simulink model "Bremsvorgang"  (R2023a)
settings: Solver=VariableStepAuto  StartTime=0.0  StopTime=10.0  RelTol=1e-3
settings Model: Creator=victoriastrobel  LastModifiedBy=victoriastrobel

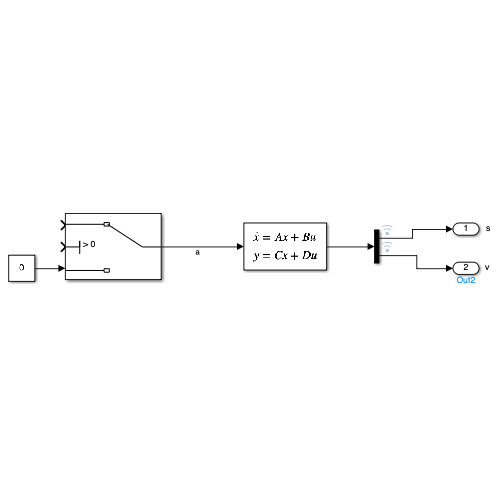
[thumbnail: Simulink's stored preview of the top-level diagram]
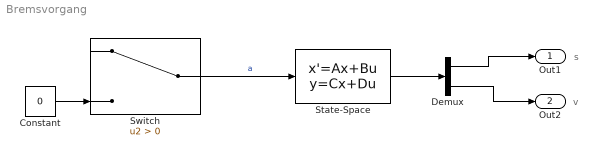
== system Bremsvorgang ==
  note: v
  note: s
  Constant : Constant  Value=0
  Demux : Demux  Outputs=2
  State-Space : StateSpace  A=[0 1; 0 0]  B=[0; 1]  C=[1 0; 0 1]  D=[0; 0]  InitialCondition=0
  Switch : Switch  Criteria=u2 > Threshold  SaturateOnIntegerOverflow=off  InputSameDT=off
  Out1 : Outport
  Out2 : Outport  Port=2
  wires:
  Constant/1 -> Switch/3
  Switch/1 -> State-Space/1  "a"
  State-Space/1 -> Demux/1
  Demux/1 -> Out1/1
  Demux/2 -> Out2/1
